simulink model "PD_controller"  (R2020a)
settings: Solver=VariableStepAuto  StartTime=0.0  StopTime=10.0  RelTol=1e-3
libraries: simulink x2
settings Model: Creator=Administrator  LastModifiedBy=Administrator

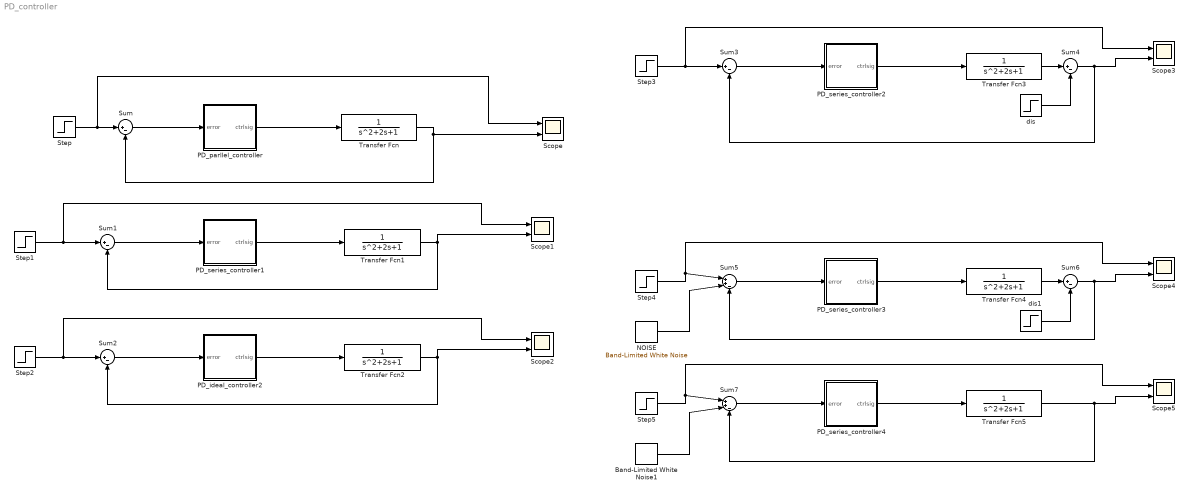
== system PD_controller ==
  Band-Limited White Noise1 : simulink/Sources/Band-Limited White Noise  Cov=[0.1]  Ts=0.1  seed=[23341]
  NOISE : simulink/Sources/Band-Limited White Noise  Cov=[0.1]  Ts=0.1  seed=[23341]
  PD_ideal_controller2 : Subsystem
  PD_parllel_controller : Subsystem
  PD_series_controller1 : Subsystem
  PD_series_controller2 : Subsystem
  PD_series_controller3 : Subsystem
  PD_series_controller4 : Subsystem
  Scope{,1..5} (6 alike) : Scope  NumInputPorts=2
  Step{,1..5} (6 alike) : Step  SampleTime=0
  Sum{,1..4,6} (6 alike) : Sum  Inputs=|+-
  Sum5 : Sum  Inputs=|++-
  Sum7 : Sum  Inputs=|++-
  Transfer Fcn{,1..5} (6 alike) : TransferFcn
  dis : Step  Time=4  SampleTime=0
  dis1 : Step  Time=4  SampleTime=0
  wires:
  Step/1 -> Scope/1, Sum/1
  dis/1 -> Sum4/2
  Transfer Fcn3/1 -> Sum4/1
  PD_series_controller2/1(ctrlsig) -> Transfer Fcn3/1
  Sum2/1 -> PD_ideal_controller2/1(error)
  Transfer Fcn2/1 -> Sum2/2, Scope2/2
  PD_series_controller1/1(ctrlsig) -> Transfer Fcn1/1
  Step3/1 -> Sum3/1, Scope3/1
  Sum3/1 -> PD_series_controller2/1(error)
  Step2/1 -> Sum2/1, Scope2/1
  Step1/1 -> Scope1/1, Sum1/1
  PD_parllel_controller/1(ctrlsig) -> Transfer Fcn/1
  Sum1/1 -> PD_series_controller1/1(error)
  Sum4/1 -> Scope3/2, Sum3/2
  PD_ideal_controller2/1(ctrlsig) -> Transfer Fcn2/1
  Sum/1 -> PD_parllel_controller/1(error)
  Transfer Fcn1/1 -> Scope1/2, Sum1/2
  Transfer Fcn/1 -> Scope/2, Sum/2
  Sum6/1 -> Sum5/3, Scope4/2
  Sum5/1 -> PD_series_controller3/1(error)
  Step4/1 -> Scope4/1, Sum5/1
  PD_series_controller3/1(ctrlsig) -> Transfer Fcn4/1
  Transfer Fcn4/1 -> Sum6/1
  dis1/1 -> Sum6/2
  NOISE/1 -> Sum5/2
  Band-Limited White Noise1/1 -> Sum7/2
  PD_series_controller4/1(ctrlsig) -> Transfer Fcn5/1
  Step5/1 -> Sum7/1, Scope5/1
  Sum7/1 -> PD_series_controller4/1(error)
  Transfer Fcn5/1 -> Scope5/2, Sum7/3

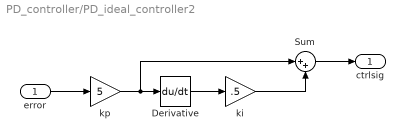
== system PD_controller/PD_ideal_controller2 ==
  error : Inport
  Derivative : Derivative
  Sum : Sum  Inputs=|++
  ki : Gain  Gain=.5
  kp : Gain  Gain=5
  ctrlsig : Outport
  wires:
  Derivative/1 -> ki/1
  ki/1 -> Sum/2
  error/1 -> kp/1
  Sum/1 -> ctrlsig/1
  kp/1 -> Derivative/1, Sum/1

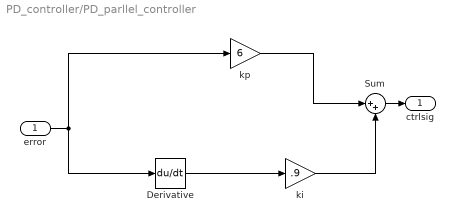
== system PD_controller/PD_parllel_controller ==
  error : Inport
  Derivative : Derivative
  Sum : Sum  Inputs=|++
  ki : Gain  Gain=.9
  kp : Gain  Gain=6
  ctrlsig : Outport
  wires:
  kp/1 -> Sum/1
  ki/1 -> Sum/2
  error/1 -> Derivative/1, kp/1
  Derivative/1 -> ki/1
  Sum/1 -> ctrlsig/1

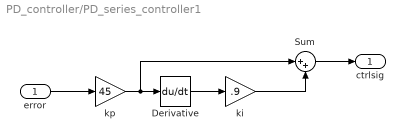
== system PD_controller/PD_series_controller1 ==
  error : Inport
  Derivative : Derivative
  Sum : Sum  Inputs=|++
  ki : Gain  Gain=.9
  kp : Gain  Gain=45
  ctrlsig : Outport
  wires:
  kp/1 -> Derivative/1, Sum/1
  Sum/1 -> ctrlsig/1
  error/1 -> kp/1
  ki/1 -> Sum/2
  Derivative/1 -> ki/1

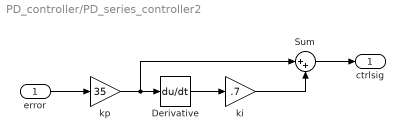
== system PD_controller/PD_series_controller2 ==
  error : Inport
  Derivative : Derivative
  Sum : Sum  Inputs=|++
  ki : Gain  Gain=.7
  kp : Gain  Gain=35
  ctrlsig : Outport
  wires:
  Derivative/1 -> ki/1
  ki/1 -> Sum/2
  error/1 -> kp/1
  Sum/1 -> ctrlsig/1
  kp/1 -> Derivative/1, Sum/1

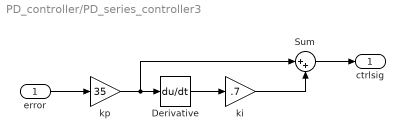
== system PD_controller/PD_series_controller3 ==
  error : Inport
  Derivative : Derivative
  Sum : Sum  Inputs=|++
  ki : Gain  Gain=.7
  kp : Gain  Gain=35
  ctrlsig : Outport
  wires:
  kp/1 -> Sum/1, Derivative/1
  Sum/1 -> ctrlsig/1
  error/1 -> kp/1
  ki/1 -> Sum/2
  Derivative/1 -> ki/1

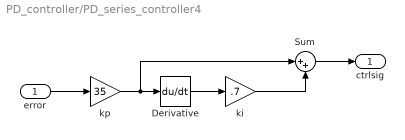
== system PD_controller/PD_series_controller4 ==
  error : Inport
  Derivative : Derivative
  Sum : Sum  Inputs=|++
  ki : Gain  Gain=.7
  kp : Gain  Gain=35
  ctrlsig : Outport
  wires:
  Derivative/1 -> ki/1
  ki/1 -> Sum/2
  error/1 -> kp/1
  Sum/1 -> ctrlsig/1
  kp/1 -> Derivative/1, Sum/1
